simulink model "Quad_UAV_Dynamics"  (R2024b)
settings: Solver=ode4  StartTime=0.0  StopTime=inf  FixedStep=SampleTime  RelTol=1e-3
PreLoadFcn:
  | InitVars;
undefined symbols (not defined in the file): contact, control, Controller, Defectiveness, Environment, Estimator, fractalcoef, m_to_mm, ms2_to_mg, ms_to_cms, Payload, ref_height, ref_lat, ref_lon, rotorDir, rotorPositions, rotorThrustMax, rotorTimeConst, rotorTorqueMax, SampleTime, SampleTimePlant, SamplingTime, Vehicle
libraries: slpidlib x9, uavmavlinklib x9, simulink_extras x3, simulink x2, sharedtransform x2, aerolibatmos2 x1, sensorgpslib x1, robotcorelib x1, mspsensorlib x1, shared6dof x1, aerolibasang x1, sldrtlib x1
(part 2 of 2)

== system Quad_UAV_Dynamics/Send Plant Feedback/HIL_QUATERNION ==
  Acc : Inport
  States : Inport  Port=2
  GPS Subsystem : Subsystem
      settings: PortSchema="{\"entries\":[{\"content\":{\"sides\":[{\"content\":{\"connectorIds\":[\"In1\"]},\"type\":\"ConnectorPlacement.EquallySpacedRectSide\",\"uuid\":\"bd7d303d-974a-4dd9-8d27-04cf87176bd7\"},{\"content\":{\"connectorIds\":[\"Out1\"],\"side\":\"RIGHT\"},\"type\":\"ConnectorPlacement.EquallySpacedRectSide\",\"uuid\":\"9b60b4cf-af27-4ca7-86b7-e75d27668f15\"},{\"content\":{\"connectorIds\":[\"In2\"],\"side\":\"TOP\"},\"type\":\"ConnectorPlacement.EquallySpacedRectSide\",\"uuid\":\"cd4d20a6-3033-4c65-942d-f02a7fa933e8\"},{\"content\":{\"side\":\"BOTTOM\"},\"type\":\"ConnectorPlacement.EquallySpacedRectSide\",\"uuid\":\"d837ff15-3ee7-4ba9-aab0-0378a7633b3a\"},{\"content\":{\"side\":\"HIDDEN\"},\"type\":\"ConnectorPlacement.EquallySpacedRectSide\",\"uuid\":\"eefe2c49-f98f-4c11-8e75-b071b558b610\"}]},\"type\":\"ConnectorPlacement.EquallySpacedConnector\",\"uuid\":\"bd9fca06-cb18-49af-bec9-4d4823ab7b04\"}],\"packageUris\":[\"http://schema.mathworks.com/mf0/Connector/R2020b\"],\"version\":\"1.0\"}"
  MAVLink Serializer2 : uavmavlinklib/MAVLink Serializer  dialectSource=Select from standard MAVLink dialects  dialect=common.xml  dialectCustom=common.xml  version=2  messageType=HIL_STATE_QUATERNION
  Terminator2 : Terminator
  HIL_QUATERNION_bytes : Outport
  wires:
  States/1 -> GPS Subsystem/1(States)
  MAVLink Serializer2/2 -> Terminator2/1
  GPS Subsystem/1(HIL Quaternion) -> MAVLink Serializer2/1
  MAVLink Serializer2/1 -> HIL_QUATERNION_bytes/1
  Acc/1 -> GPS Subsystem/2(Acc)

== system Quad_UAV_Dynamics/Send Plant Feedback/HIL_SENSOR ==
  Acc : Inport
  Gyro : Inport  Port=2
  Mag : Inport  Port=3
  Pressure : Inport  Port=4
  Hil Sensor Creation subsystem : Subsystem
  MAVLink Serializer1 : uavmavlinklib/MAVLink Serializer  dialectSource=Select from standard MAVLink dialects  dialect=common.xml  dialectCustom=common.xml  version=2  messageType=HIL_SENSOR
  Terminator1 : Terminator
  HIL_SENSOR_bytes : Outport
  wires:
  MAVLink Serializer1/2 -> Terminator1/1
  Hil Sensor Creation subsystem/1(HIL Sensor) -> MAVLink Serializer1/1
  Acc/1 -> Hil Sensor Creation subsystem/1(Acc)
  MAVLink Serializer1/1 -> HIL_SENSOR_bytes/1
  Gyro/1 -> Hil Sensor Creation subsystem/2(Gyro)
  Mag/1 -> Hil Sensor Creation subsystem/3(Mag)
  Pressure/1 -> Hil Sensor Creation subsystem/4(Pressure)

== system Quad_UAV_Dynamics/Send Plant Feedback/Send Heartbeat ==
  Bus Assignment : BusAssignment  AssignedSignals=Payload.autopilot,Payload.type
  Constant : Constant  SampleTime=-1
  Constant1 : Constant  Value=12  SampleTime=-1
  Data Type Conversion : DataTypeConversion  OutDataTypeStr=uint8  SaturateOnIntegerOverflow=off  RndMeth=Floor
  Data Type Conversion1 : DataTypeConversion  OutDataTypeStr=uint8  SaturateOnIntegerOverflow=off  RndMeth=Floor
  MAVLink Blank Message : uavmavlinklib/MAVLink Blank Message  dialectSource=Select from standard MAVLink dialects  dialect=common.xml  dialectCustom=common.xml  version=2  messageType=HEARTBEAT  SystemID=2  ComponentID=51  SampleTime=SampleTime
  MAVLink Serializer : uavmavlinklib/MAVLink Serializer  dialectSource=Select from standard MAVLink dialects  dialect=common.xml  dialectCustom=common.xml  version=2  messageType=HEARTBEAT
  Terminator4 : Terminator
  HEARTBEAT_bytes : Outport
  wires:
  Bus Assignment/1 -> MAVLink Serializer/1
  Constant/1 -> Data Type Conversion/1
  MAVLink Serializer/1 -> HEARTBEAT_bytes/1
  Data Type Conversion1/1 -> Bus Assignment/3
  Data Type Conversion/1 -> Bus Assignment/2
  MAVLink Serializer/2 -> Terminator4/1
  Constant1/1 -> Data Type Conversion1/1
  MAVLink Blank Message/1 -> Bus Assignment/1

== system Quad_UAV_Dynamics/Plant/IMU Simulation/IMU Subsystem ==
  States : Inport
  Bus Selector1 : BusSelector  OutputSignals=p,q,r  OutputAsBus=on
  Bus Selector2 : BusSelector  OutputSignals=yaw,pitch,roll  OutputAsBus=on
  Bus Selector3 : BusSelector  OutputSignals=ddx,ddy,ddz  OutputAsBus=on
  Coordinate Transformation Conversion1 : robotcorelib/Coordinate Transformation Conversion  InputRepresentation=Euler Angles  InputEulerSequence=ZYX  ShowTrVecInputPort=on  OutputRepresentation=Quaternion  OutputEulerSequence=ZYX  ShowTrVecOutputPort=on  SimulateUsing=Interpreted execution
  Gain : Gain  Gain=-1
  IMU : mspsensorlib/IMU  DispRefFrame=NED  TemperaturePort=off  Temperature=25  MagneticFieldPort=off  MagneticFieldNED=[ 27.5550, -2.4169, -16.0849 ]  MagneticFieldENU=[ -2.4169, 27.5550, 16.0849 ]  SeedDouble=67  SimulateUsing=Interpreted execution  AccelParamsMeasurementRange=Inf  AccelParamsResolution=0  AccelParamsConstantBias=[ 0, 0, 0 ]  AccelParamsAxesMisalignment=[ 0, 0, 0 ]  AccelParamsNoiseDensity=[ 0, 0, 0 ]  AccelParamsBiasInstability=[ 0, 0, 0 ]  AccelParamsBiasInstabilityNumerator=fractalcoef().Numerator  AccelParamsBiasInstabilityDenominator=fractalcoef().Denominator  AccelParamsRandomWalk=[ 0, 0, 0 ]  AccelParamsNoiseType=double-sided  AccelParamsTemperatureBias=[ 0, 0, 0 ]  AccelParamsTemperatureScaleFactor=[ 0, 0, 0 ]  GyroParamsMeasurementRange=Inf  GyroParamsResolution=0  GyroParamsConstantBias=[ 0, 0, 0 ]  GyroParamsAxesMisalignment=[ 0, 0, 0 ]  GyroParamsAccelerationBias=[ 0, 0, 0 ]  GyroParamsNoiseDensity=[ 0, 0, 0 ]  GyroParamsBiasInstability=[ 0, 0, 0 ]  GyroParamsBiasInstabilityNumerator=fractalcoef().Numerator  GyroParamsBiasInstabilityDenominator=fractalcoef().Denominator  GyroParamsRandomWalk=[ 0, 0, 0 ]  GyroParamsNoiseType=double-sided  GyroParamsTemperatureBias=[ 0, 0, 0 ]  GyroParamsTemperatureScaleFactor=[ 0, 0, 0 ]  MagParamsMeasurementRange=Inf  MagParamsResolution=0  MagParamsConstantBias=[ 0, 0, 0 ]  MagParamsAxesMisalignment=[ 0, 0, 0 ]  MagParamsNoiseDensity=[ 0, 0, 0 ]  MagParamsBiasInstability=[ 0, 0, 0 ]  MagParamsBiasInstabilityNumerator=fractalcoef().Numerator  MagParamsBiasInstabilityDenominator=fractalcoef().Denominator  MagParamsRandomWalk=[ 0, 0, 0 ]  MagParamsNoiseType=double-sided  MagParamsTemperatureBias=[ 0, 0, 0 ]  MagParamsTemperatureScaleFactor=[ 0, 0, 0 ]
  Reshape : Reshape  OutputDimensionality=Row vector (2-D)
  Reshape2 : Reshape  OutputDimensionality=Row vector (2-D)
  Reshape3 : Reshape  OutputDimensionality=Row vector (2-D)
  Acc : Outport
  Gyro : Outport  Port=2
  Mag : Outport  Port=3
  wires:
  Bus Selector1/1 -> Reshape2/1
  IMU/1 -> Gain/1
  Bus Selector2/1 -> Coordinate Transformation Conversion1/1
  IMU/3 -> Mag/1
  Reshape2/1 -> IMU/2
  Bus Selector3/1 -> Reshape/1
  Coordinate Transformation Conversion1/1 -> Reshape3/1
  Reshape/1 -> IMU/1
  IMU/2 -> Gyro/1
  Reshape3/1 -> IMU/3
  States/1 -> Bus Selector3/1, Bus Selector2/1, Bus Selector1/1
  Gain/1 -> Acc/1

== system Quad_UAV_Dynamics/Plant/Non-Linear Airframe/AC model ==
  Actuators : Inport
  States : Inport  Port=2
  Add1 : Sum  Inputs=++++
  Add2 : Sum  Inputs=+++
  Aerodynamic : Subsystem
  Bus Selector3 : BusSelector  OutputSignals=DCM
  Constant : Constant  Value=Environment.g
  Constant1 : Constant  Value=Environment.rho
  Gravity Force Calculation : Subsystem
  Ground Model : Subsystem
  Motor Forces and Torques : Subsystem
  Rotor Model : Subsystem  Commented=on
  F_cg : Outport  Unit=N  VectorParamsAs1DForOutWhenUnconnected=off
  M_cg : Outport  Port=2  Unit=N*m  VectorParamsAs1DForOutWhenUnconnected=off
  wires:
  Add1/1 -> F_cg/1
  Constant/1 -> Gravity Force Calculation/2(gravity)
  Constant1/1 -> Aerodynamic/1(Density)
  States/1 -> Bus Selector3/1, Ground Model/1(States), Aerodynamic/2(States)
  Actuators/1 -> Motor Forces and Torques/1(Input [0-1])
  Bus Selector3/1 -> Gravity Force Calculation/1(DCMbe)  "<DCM>"
  Add2/1 -> M_cg/1
  Motor Forces and Torques/2(Motor Torques) -> Add2/2
  Motor Forces and Torques/1(Motor Forces) -> Add1/3
  Gravity Force Calculation/1(gravity force) -> Add1/1
  Aerodynamic/2(Moment) -> Add2/1
  Aerodynamic/1(Force) -> Add1/2
  Ground Model/1(Fb_contact) -> Add1/4
  Ground Model/2(Mb_contact) -> Add2/3

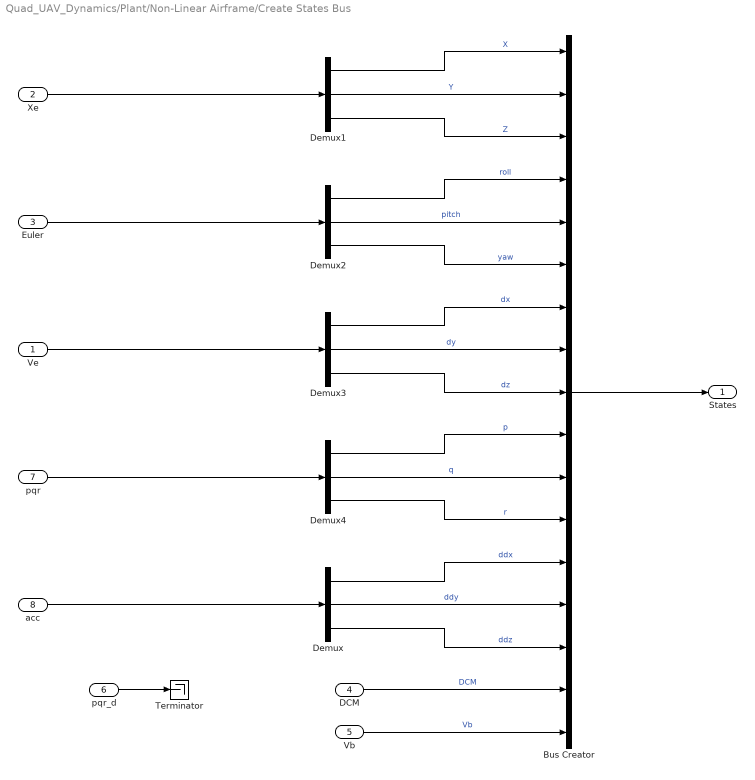
== system Quad_UAV_Dynamics/Plant/Non-Linear Airframe/Create States Bus ==
  Ve : Inport
  Xe : Inport  Port=2
  Euler : Inport  Port=3
  DCM : Inport  Port=4
  Vb : Inport  Port=5
  pqr_d : Inport  Port=6
  pqr : Inport  Port=7
  acc : Inport  Port=8
  Bus Creator : BusCreator  Inputs=17
  Demux{,1..4} (5 alike) : Demux  Outputs=3
  Terminator : Terminator
  States : Outport
  wires:
  Demux1/1 -> Bus Creator/1  "X"
  Demux1/2 -> Bus Creator/2  "Y"
  Euler/1 -> Demux2/1
  Demux2/2 -> Bus Creator/5  "pitch"
  Demux3/2 -> Bus Creator/8  "dy"
  Demux2/3 -> Bus Creator/6  "yaw"
  pqr/1 -> Demux4/1
  Ve/1 -> Demux3/1
  Demux2/1 -> Bus Creator/4  "roll"
  Demux1/3 -> Bus Creator/3  "Z"
  Demux3/1 -> Bus Creator/7  "dx"
  Demux4/2 -> Bus Creator/11  "q"
  Demux3/3 -> Bus Creator/9  "dz"
  Demux4/3 -> Bus Creator/12  "r"
  Demux4/1 -> Bus Creator/10  "p"
  Bus Creator/1 -> States/1
  Xe/1 -> Demux1/1
  acc/1 -> Demux/1
  Demux/3 -> Bus Creator/15  "ddz"
  Demux/2 -> Bus Creator/14  "ddy"
  Demux/1 -> Bus Creator/13  "ddx"
  DCM/1 -> Bus Creator/16  "DCM"
  Vb/1 -> Bus Creator/17  "Vb"
  pqr_d/1 -> Terminator/1

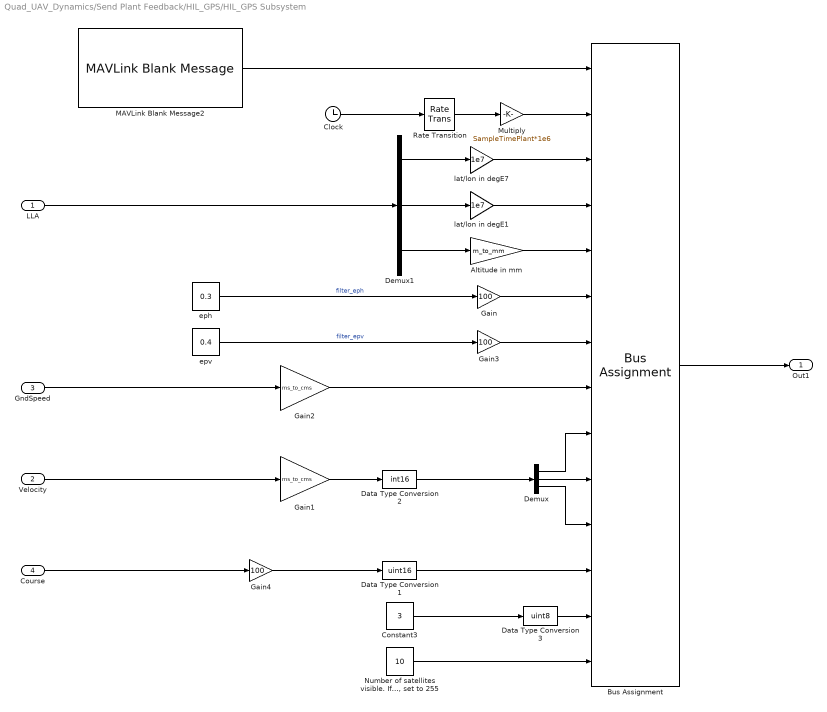
== system Quad_UAV_Dynamics/Send Plant Feedback/HIL_GPS/HIL_GPS Subsystem ==
  LLA : Inport
  Velocity : Inport  Port=2
  GndSpeed : Inport  Port=3
  Course : Inport  Port=4
  Altitude in mm : Gain  Gain=m_to_mm  OutDataTypeStr=Inherit: Inherit via back propagation
  Bus Assignment : BusAssignment  AssignedSignals=Payload.time_usec,Payload.lat,Payload.lon,Payload.alt,Payload.eph,Payload.epv,Payload.vel,Payload.vn,Payload.ve,Payload.vd,Payload.cog,Payload.fix_type,Payload.satellites_visible
  Clock : Clock
  Constant3 : Constant  Value=3  OutDataTypeStr=Inherit: Inherit via back propagation  SampleTime=-1
  Data Type Conversion1 : DataTypeConversion  OutDataTypeStr=uint16  SaturateOnIntegerOverflow=off  RndMeth=Floor
  Data Type Conversion2 : DataTypeConversion  OutDataTypeStr=int16  SaturateOnIntegerOverflow=off  RndMeth=Floor
  Data Type Conversion3 : DataTypeConversion  OutDataTypeStr=uint8  SaturateOnIntegerOverflow=off  RndMeth=Floor
  Demux : Demux  Outputs=3
  Demux1 : Demux  Outputs=3
  Gain : Gain  Gain=100  OutDataTypeStr=Inherit: Inherit via back propagation
  Gain1 : Gain  Gain=ms_to_cms
  Gain2 : Gain  Gain=ms_to_cms  OutDataTypeStr=uint16
  Gain3 : Gain  Gain=100  OutDataTypeStr=Inherit: Inherit via back propagation
  Gain4 : Gain  Gain=100
  MAVLink Blank Message2 : uavmavlinklib/MAVLink Blank Message  dialectSource=Select from standard MAVLink dialects  dialect=common.xml  dialectCustom=common.xml  version=2  messageType=HIL_GPS  SystemID=2  ComponentID=51  SampleTime=SampleTime
  Multiply : Gain  Gain=SampleTimePlant*1e6  OutDataTypeStr=Inherit: Inherit via back propagation
  "Number of satellites visible. If unknown, set to 255" : Constant  Value=10  OutDataTypeStr=Inherit: Inherit via back propagation  SampleTime=-1
  Rate Transition : RateTransition
  eph : Constant  Value=0.3  SampleTime=-1
  epv : Constant  Value=0.4  SampleTime=-1
  lat/lon in degE1 : Gain  Gain=1e7  OutDataTypeStr=Inherit: Inherit via back propagation
  lat/lon in degE7 : Gain  Gain=1e7  OutDataTypeStr=Inherit: Inherit via back propagation
  Out1 : Outport
  wires:
  Gain2/1 -> Bus Assignment/8
  lat/lon in degE7/1 -> Bus Assignment/3
  Demux1/1 -> lat/lon in degE7/1
  Demux/3 -> Bus Assignment/11
  MAVLink Blank Message2/1 -> Bus Assignment/1
  Gain1/1 -> Data Type Conversion2/1
  Demux1/3 -> Altitude in mm/1
  Demux1/2 -> lat/lon in degE1/1
  Demux/1 -> Bus Assignment/9
  lat/lon in degE1/1 -> Bus Assignment/4
  Altitude in mm/1 -> Bus Assignment/5
  Data Type Conversion2/1 -> Demux/1
  Demux/2 -> Bus Assignment/10
  Bus Assignment/1 -> Out1/1
  "Number of satellites visible. If unknown, set to 255"/1 -> Bus Assignment/14
  Gain/1 -> Bus Assignment/6
  Gain3/1 -> Bus Assignment/7
  LLA/1 -> Demux1/1
  GndSpeed/1 -> Gain2/1
  Velocity/1 -> Gain1/1
  Course/1 -> Gain4/1
  Data Type Conversion1/1 -> Bus Assignment/12
  eph/1 -> Gain/1  "filter_eph"
  epv/1 -> Gain3/1  "filter_epv"
  Data Type Conversion3/1 -> Bus Assignment/13
  Gain4/1 -> Data Type Conversion1/1
  Constant3/1 -> Data Type Conversion3/1
  Clock/1 -> Rate Transition/1
  Rate Transition/1 -> Multiply/1
  Multiply/1 -> Bus Assignment/2

== system Quad_UAV_Dynamics/Send Plant Feedback/HIL_QUATERNION/GPS Subsystem ==
  States : Inport
  Acc : Inport  Port=2
  HIL Quaternion Creation Subsystem : Subsystem
  HIL Quaternion : Outport
  wires:
  HIL Quaternion Creation Subsystem/1(HIL Quaternion) -> HIL Quaternion/1
  States/1 -> HIL Quaternion Creation Subsystem/2(States)
  Acc/1 -> HIL Quaternion Creation Subsystem/1(Acc)

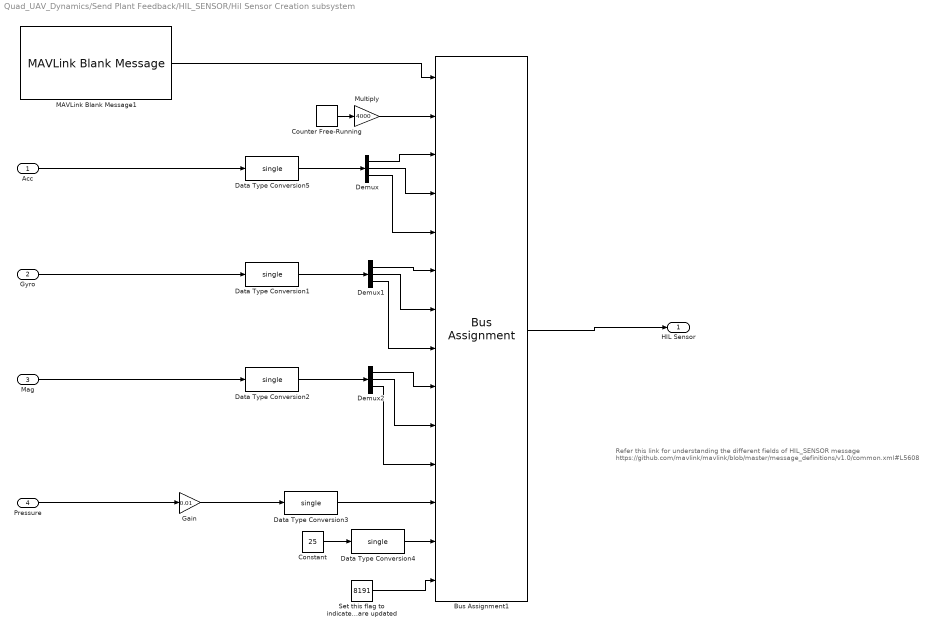
== system Quad_UAV_Dynamics/Send Plant Feedback/HIL_SENSOR/Hil Sensor Creation subsystem ==
  note: Refer this link for understanding the different fields of HIL_SENSOR message https://github.com/mavlink/mavlink/blob/master/message_definitions/v1.0/common.xml#L5608
  Acc : Inport
  Gyro : Inport  Port=2
  Mag : Inport  Port=3
  Pressure : Inport  Port=4
  Bus Assignment1 : BusAssignment  AssignedSignals=Payload.time_usec,Payload.xacc,Payload.yacc,Payload.zacc,Payload.xgyro,Payload.ygyro,Payload.zgyro,Payload.xmag,Payload.ymag,Payload.zmag,Payload.abs_pressure,Payload.temperature,Payload.fields_updated
  Constant : Constant  Value=25
  Counter Free-Running : simulink/Sources/Counter Free-Running  NumBits=64  tsamp=SampleTime
  Data Type Conversion{1..5} (5 alike) : DataTypeConversion  OutDataTypeStr=single  SaturateOnIntegerOverflow=off  RndMeth=Floor
  Demux : Demux  Outputs=3
  Demux1 : Demux  Outputs=3
  Demux2 : Demux  Outputs=3
  Gain : Gain  Gain=0.01
  MAVLink Blank Message1 : uavmavlinklib/MAVLink Blank Message  dialectSource=Select from standard MAVLink dialects  dialect=common.xml  dialectCustom=common.xml  version=2  messageType=HIL_SENSOR  SystemID=2  ComponentID=51  SampleTime=SampleTime
  Multiply : Gain  Gain=4000  OutDataTypeStr=Inherit: Inherit via back propagation
  Set this flag to indicate all flags are updated : Constant  Value=8191  OutDataTypeStr=Inherit: Inherit via back propagation  SampleTime=-1
  HIL Sensor : Outport
  wires:
  Data Type Conversion2/1 -> Demux2/1
  Demux1/1 -> Bus Assignment1/6
  Counter Free-Running/1 -> Multiply/1
  Demux1/3 -> Bus Assignment1/8
  Data Type Conversion1/1 -> Demux1/1
  Gyro/1 -> Data Type Conversion1/1
  Bus Assignment1/1 -> HIL Sensor/1
  Set this flag to indicate all flags are updated/1 -> Bus Assignment1/14
  Demux/3 -> Bus Assignment1/5
  Demux2/2 -> Bus Assignment1/10
  Demux2/3 -> Bus Assignment1/11
  Data Type Conversion5/1 -> Demux/1
  Demux/1 -> Bus Assignment1/3
  MAVLink Blank Message1/1 -> Bus Assignment1/1
  Demux2/1 -> Bus Assignment1/9
  Demux/2 -> Bus Assignment1/4
  Demux1/2 -> Bus Assignment1/7
  Acc/1 -> Data Type Conversion5/1
  Mag/1 -> Data Type Conversion2/1
  Data Type Conversion3/1 -> Bus Assignment1/12
  Gain/1 -> Data Type Conversion3/1
  Pressure/1 -> Gain/1
  Constant/1 -> Data Type Conversion4/1
  Data Type Conversion4/1 -> Bus Assignment1/13
  Multiply/1 -> Bus Assignment1/2

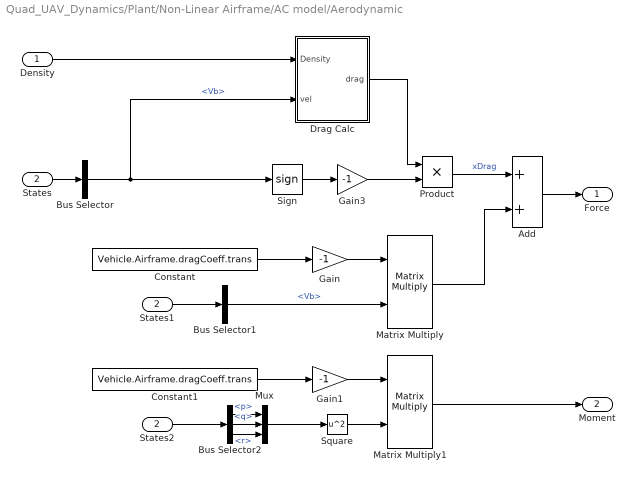
== system Quad_UAV_Dynamics/Plant/Non-Linear Airframe/AC model/Aerodynamic ==
  Density : Inport  Unit=kg/m^3
  States : Inport  Port=2
  Add : Sum
  Bus Selector : BusSelector  OutputSignals=Vb
  Bus Selector1 : BusSelector  OutputSignals=Vb
  Bus Selector2 : BusSelector  OutputSignals=p,q,r
  Constant : Constant  Value=Vehicle.Airframe.dragCoeff.trans
  Constant1 : Constant  Value=Vehicle.Airframe.dragCoeff.trans
  Drag Calc : Subsystem
  Gain : Gain  Gain=-1
  Gain1 : Gain  Gain=-1
  Gain3 : Gain  Gain=-1
  Matrix Multiply : Product  Multiplication=Matrix(*)
  Matrix Multiply1 : Product  Multiplication=Matrix(*)
  Mux : Mux  Inputs=3
  Product : Product  RndMeth=Zero
  Sign : Signum  ZeroCross=off
  Square : Math  Operator=square
  States1 : InportShadow  Port=2
  States2 : InportShadow  Port=2
  Force : Outport  Unit=N  VectorParamsAs1DForOutWhenUnconnected=off
  Moment : Outport  Port=2  Unit=N  VectorParamsAs1DForOutWhenUnconnected=off
  wires:
  Density/1 -> Drag Calc/1(Density)
  Sign/1 -> Gain3/1
  Drag Calc/1(drag) -> Product/1
  Product/1 -> Add/1  "xDrag"
  Bus Selector/1 -> Drag Calc/2(vel), Sign/1  "<Vb>"
  Gain3/1 -> Product/2
  States/1 -> Bus Selector/1
  Constant/1 -> Gain/1
  States1/1 -> Bus Selector1/1
  Bus Selector1/1 -> Matrix Multiply/2  "<Vb>"
  Matrix Multiply/1 -> Add/2
  Add/1 -> Force/1
  Constant1/1 -> Gain1/1
  States2/1 -> Bus Selector2/1
  Gain/1 -> Matrix Multiply/1
  Gain1/1 -> Matrix Multiply1/1
  Square/1 -> Matrix Multiply1/2
  Matrix Multiply1/1 -> Moment/1
  Bus Selector2/1 -> Mux/1  "<p>"
  Bus Selector2/2 -> Mux/2  "<q>"
  Bus Selector2/3 -> Mux/3  "<r>"
  Mux/1 -> Square/1

== system Quad_UAV_Dynamics/Plant/Non-Linear Airframe/AC model/Gravity Force Calculation ==
  DCMbe : Inport
  gravity : Inport  Port=2  Unit=m/s^2
  Gain1 : Gain  Gain=Vehicle.Airframe.mass
  Product : Product  Multiplication=Matrix(*)
  gravity force : Outport  Unit=N  VectorParamsAs1DForOutWhenUnconnected=off
  wires:
  gravity/1 -> Gain1/1
  Gain1/1 -> Product/2  "gravity force NED"
  Product/1 -> gravity force/1
  DCMbe/1 -> Product/1

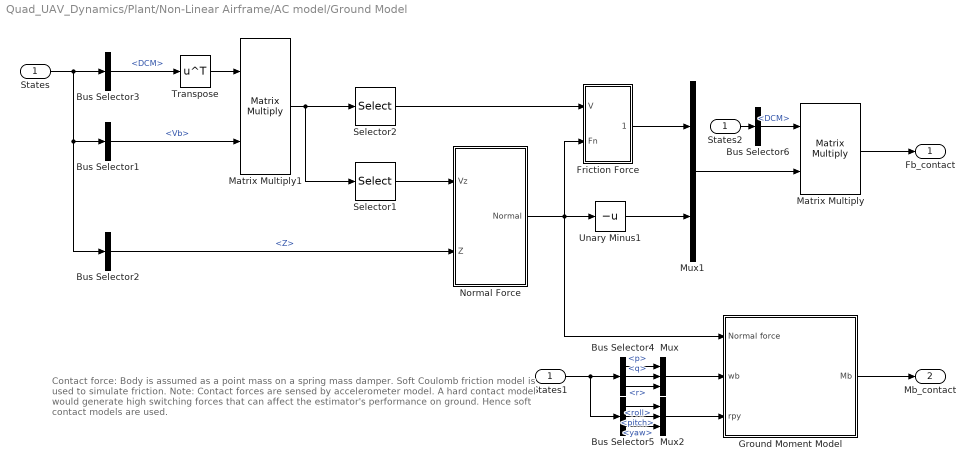
== system Quad_UAV_Dynamics/Plant/Non-Linear Airframe/AC model/Ground Model ==
  note: Contact force:
      | Body is assumed as a point mass on a spring mass damper. Soft Coulomb friction model is used to simulate friction.
      |
      | Note:
      | Contact forces are sensed by accelerometer model. A hard contact model would generate high switching forces that can affect the estimator's performance on ground. Hence soft contact models are used.
  States : Inport
  Bus Selector1 : BusSelector  OutputSignals=Vb
  Bus Selector2 : BusSelector  OutputSignals=Z
  Bus Selector3 : BusSelector  OutputSignals=DCM
  Bus Selector4 : BusSelector  OutputSignals=p,q,r
  Bus Selector5 : BusSelector  OutputSignals=roll,pitch,yaw
  Bus Selector6 : BusSelector  OutputSignals=DCM
  Friction Force : Subsystem
  Ground Moment Model : Subsystem
  Matrix Multiply : Product  Multiplication=Matrix(*)
  Matrix Multiply1 : Product  Multiplication=Matrix(*)
  Mux : Mux  Inputs=3
  Mux1 : Mux  Inputs=2
  Mux2 : Mux  Inputs=3
  Normal Force : Subsystem
  Selector1 : Selector  InputPortWidth=3  IndexOptions=Index vector (dialog)  Indices=[3]  OutputSizes=1
  Selector2 : Selector  InputPortWidth=3  IndexOptions=Index vector (dialog)  Indices=[1,2]  OutputSizes=1
  States1 : InportShadow
  States2 : InportShadow
  Transpose : Math  Operator=transpose
  Unary Minus1 : UnaryMinus
  Fb_contact : Outport
  Mb_contact : Outport  Port=2
  wires:
  Selector1/1 -> Normal Force/1(Vz)
  Bus Selector2/1 -> Normal Force/2(Z)  "<Z>"
  Matrix Multiply/1 -> Fb_contact/1
  Normal Force/1(Normal) -> Unary Minus1/1, Ground Moment Model/1(Normal force), Friction Force/2(Fn)
  Mux1/1 -> Matrix Multiply/2
  Unary Minus1/1 -> Mux1/2
  Selector2/1 -> Friction Force/1(V)
  Friction Force/1(Friction) -> Mux1/1
  Bus Selector3/1 -> Transpose/1  "<DCM>"
  Transpose/1 -> Matrix Multiply1/1
  Bus Selector1/1 -> Matrix Multiply1/2  "<Vb>"
  Matrix Multiply1/1 -> Selector1/1, Selector2/1
  Ground Moment Model/1(Mb) -> Mb_contact/1
  States/1 -> Bus Selector3/1, Bus Selector1/1, Bus Selector2/1
  States1/1 -> Bus Selector4/1, Bus Selector5/1
  Bus Selector4/1 -> Mux/1  "<p>"
  Bus Selector4/2 -> Mux/2  "<q>"
  Bus Selector4/3 -> Mux/3  "<r>"
  Mux/1 -> Ground Moment Model/2(wb)
  Bus Selector5/1 -> Mux2/1  "<roll>"
  Bus Selector5/2 -> Mux2/2  "<pitch>"
  Bus Selector5/3 -> Mux2/3  "<yaw>"
  Mux2/1 -> Ground Moment Model/3(rpy)
  States2/1 -> Bus Selector6/1
  Bus Selector6/1 -> Matrix Multiply/1  "<DCM>"

== system Quad_UAV_Dynamics/Plant/Non-Linear Airframe/AC model/Motor Forces and Torques ==
  Input [0-1] : Inport
  Add : Sum
  Deffectiveness : Subsystem  Commented=on  mask(Control Signal Mapper){d1=Defectiveness.Actuator_1.value, d2=Defectiveness.Actuator_2.value, d3=Defectiveness.Actuator_3.value, d4=Defectiveness.Actuator_4.value, d1_start=Defectiveness.Actuator_1.StartTime, d1_stop=Defectiveness.Actuator_1.endTime, d2_start=Defectiveness.Actuator_2.StartTime, d2_stop=Defectiveness.Actuator_2.endTime, d3_start=Defectiveness.Actuator_3.StartTime, d3_stop=Defectiveness.Actuator_3.endTime, d4_start=Defectiveness.Actuator_4.StartTime, d4_stop=Defectiveness.Actuator_4.endTime}
      mask prompts: d1 "Actuator-1"; d2 "Actuator-2"; d3 "Actuator-3"; d4 "Actuator-4"; d1_start "Start"; d1_stop "Stop"; d2_start "Start"; d2_stop "Stop"; d3_start "Start"; d3_stop "Stop"; d4_start "Start"; d4_stop "Stop"
      mask help:
      | This block maps control signals to each actuator. This block also generates a desired defectiveness value at specified start and stop time.
      |
      | Minimum and maximum defectiveness values are 0 and 1 respectively.
      settings: MinAlgLoopOccurrences=on
      mask Help: Should user exceeds the max or min value the limitation will correct it.
      mask DialogControl ParameterGroupVar Prompt: Defectiveness Values
      mask DialogControl Container4 Prompt: Defectiveness Time
      mask DialogControl Container5 Prompt: Actuator - 1
      mask DialogControl Container6 Prompt: Actuator - 2
      mask DialogControl Container8 Prompt: Actuator - 3
      mask DialogControl Container9 Prompt: Actuator - 4
  Gain2 : Gain  Gain=-1
  Gyroscopic Moments : Subsystem
  Mapper : Constant  Value=Controller.motorMapper  OutDataTypeStr=double
  Motor : Subsystem
  Mux : Mux  Inputs=3
  Product : Product  Multiplication=Matrix(*)  RndMeth=Zero
  Selector : Selector  InputPortWidth=4  IndexOptions=Index vector (dialog)  Indices=1  OutputSizes=1
  Selector1 : Selector  InputPortWidth=4  IndexOptions=Index vector (dialog)  Indices=2:4  OutputSizes=1
  Square : Math  Operator=square
  Zero : Constant  Value=0  OutDataTypeStr=Inherit: Inherit via back propagation
  Motor Forces : Outport  OutDataTypeStr=double  Unit=N  PortDimensions=3  SampleTime=0  VectorParamsAs1DForOutWhenUnconnected=off
  Motor Torques : Outport  Port=2  OutDataTypeStr=double  Unit=N*m  PortDimensions=3  SampleTime=0  VectorParamsAs1DForOutWhenUnconnected=off
  wires:
  Square/1 -> Product/2
  Gyroscopic Moments/1(M) -> Add/2
  Add/1 -> Motor Torques/1
  Motor/1(rpm) -> Square/1, Gyroscopic Moments/1(Omega)
  Input [0-1]/1 -> Motor/1(PWM)
  Product/1 -> Selector1/1, Selector/1
  Gain2/1 -> Motor Forces/1
  Selector/1 -> Mux/3
  Mapper/1 -> Product/1
  Selector1/1 -> Add/1
  Mux/1 -> Gain2/1
  Zero/1 -> Mux/2, Mux/1

== system Quad_UAV_Dynamics/Plant/Non-Linear Airframe/AC model/Rotor Model ==
  Input [0-1] : Inport
  Constant : Constant  Value=rotorPositions
  Constant1 : Constant  Value=rotorDir
  MATLAB Function : MATLAB Function  TreatAsAtomicUnit=on
  Thrust model : Subsystem
  Torque model : Subsystem
  F_rotors : Outport
  M_rotors : Outport  Port=2
  wires:
  Input [0-1]/1 -> Torque model/1(In1), Thrust model/1(In1)
  MATLAB Function/1(netF) -> F_rotors/1
  MATLAB Function/2(netM) -> M_rotors/1
  Constant/1 -> MATLAB Function/3(rotorPositions)
  Constant1/1 -> MATLAB Function/4(rotorDir)
  Torque model/1(Out1) -> MATLAB Function/2(tauEachRotor)
  Thrust model/1(Out1) -> MATLAB Function/1(thrustEachRotor)

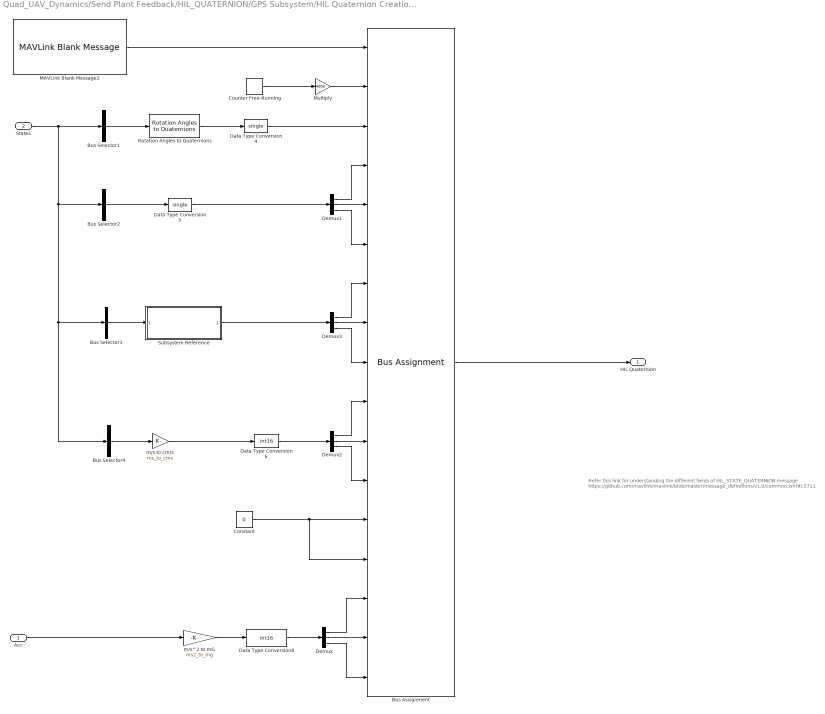
== system Quad_UAV_Dynamics/Send Plant Feedback/HIL_QUATERNION/GPS Subsystem/HIL Quaternion Creation Subsystem ==
  note: Refer this link for understanding the different fields of HIL_STATE_QUATERNION message https://github.com/mavlink/mavlink/blob/master/message_definitions/v1.0/common.xml#L5711
  Acc : Inport
  States : Inport  Port=2
  Bus Assignment : BusAssignment  AssignedSignals=Payload.time_usec,Payload.attitude_quaternion,Payload.rollspeed,Payload.pitchspeed,Payload.yawspeed,Payload.lat,Payload.lon,Payload.alt,Payload.vx,Payload.vy,Payload.vz,Payload.ind_airspeed,Payload.true_airspeed,Payload.xacc,Payload.yacc,Payload.zacc
  Bus Selector1 : BusSelector  OutputSignals=yaw,pitch,roll  OutputAsBus=on
  Bus Selector2 : BusSelector  OutputSignals=r,q,p  OutputAsBus=on
  Bus Selector3 : BusSelector  OutputSignals=X,Y,Z  OutputAsBus=on
  Bus Selector4 : BusSelector  OutputSignals=dx,dy,dz  OutputAsBus=on
  Constant : Constant  Value=0  OutDataTypeStr=Inherit: Inherit via back propagation
  Counter Free-Running : simulink/Sources/Counter Free-Running  NumBits=64  tsamp=-1
  Data Type Conversion4 : DataTypeConversion  OutDataTypeStr=single  SaturateOnIntegerOverflow=off  RndMeth=Floor
  Data Type Conversion5 : DataTypeConversion  OutDataTypeStr=single  SaturateOnIntegerOverflow=off  RndMeth=Floor
  Data Type Conversion6 : DataTypeConversion  OutDataTypeStr=int16  SaturateOnIntegerOverflow=off  RndMeth=Floor
  Data Type Conversion8 : DataTypeConversion  OutDataTypeStr=int16  SaturateOnIntegerOverflow=off  RndMeth=Floor
  Demux{,1..3} (4 alike) : Demux  Outputs=3
  MAVLink Blank Message2 : uavmavlinklib/MAVLink Blank Message  dialectSource=Select from standard MAVLink dialects  dialect=common.xml  dialectCustom=common.xml  version=2  messageType=HIL_STATE_QUATERNION  SystemID=2  ComponentID=51  SampleTime=SampleTime
  Multiply : Gain  Gain=4000  OutDataTypeStr=Inherit: Inherit via back propagation
  Rotation Angles to Quaternions : sharedtransform/Rotation Angles to Quaternions  rotationOrder=ZYX  aMode=aMode
  Subsystem Reference : Subsystem  ReferencedSubsystem=Create_LLA_from_States
  m/s to cm/s : Gain  Gain=ms_to_cms
  m/s^2 to mG : Gain  Gain=ms2_to_mg
  HIL Quaternion : Outport
  wires:
  Counter Free-Running/1 -> Multiply/1
  MAVLink Blank Message2/1 -> Bus Assignment/1
  Multiply/1 -> Bus Assignment/2
  Bus Assignment/1 -> HIL Quaternion/1
  States/1 -> Bus Selector1/1, Bus Selector2/1, Bus Selector4/1, Bus Selector3/1
  Rotation Angles to Quaternions/1 -> Data Type Conversion4/1
  Data Type Conversion4/1 -> Bus Assignment/3
  Demux/3 -> Bus Assignment/17
  Demux/1 -> Bus Assignment/15
  Demux/2 -> Bus Assignment/16
  Constant/1 -> Bus Assignment/14, Bus Assignment/13
  m/s to cm/s/1 -> Data Type Conversion6/1
  Data Type Conversion6/1 -> Demux2/1
  Demux2/3 -> Bus Assignment/12
  Demux2/2 -> Bus Assignment/11
  Demux2/1 -> Bus Assignment/10
  Subsystem Reference/1 -> Demux3/1
  Demux3/1 -> Bus Assignment/7
  Demux3/2 -> Bus Assignment/8
  Demux3/3 -> Bus Assignment/9
  Data Type Conversion8/1 -> Demux/1
  Acc/1 -> m/s^2 to mG/1
  m/s^2 to mG/1 -> Data Type Conversion8/1
  Bus Selector1/1 -> Rotation Angles to Quaternions/1
  Data Type Conversion5/1 -> Demux1/1
  Demux1/3 -> Bus Assignment/6
  Demux1/2 -> Bus Assignment/5
  Demux1/1 -> Bus Assignment/4
  Bus Selector2/1 -> Data Type Conversion5/1
  Bus Selector3/1 -> Subsystem Reference/1
  Bus Selector4/1 -> m/s to cm/s/1

== system Quad_UAV_Dynamics/Plant/Non-Linear Airframe/AC model/Aerodynamic/Drag Calc ==
  Density : Inport  Unit=kg/m^3
  vel : Inport  Port=2  Unit=m/s
  Dynamic Pressure : aerolibasang/Dynamic Pressure
  Heigth : Gain  Gain=0.1
  Mux1 : Mux  Inputs=3
  Product : Product  Inputs=3  RndMeth=Zero
  Square : Math  Operator=square
  diameter : Constant  Value=Vehicle.Airframe.armLength*sqrt(2)  SampleTime=0
  dragCoeff : Constant  Value=Vehicle.Airframe.Cdx  SampleTime=0
  drag : Outport  Unit=N  VectorParamsAs1DForOutWhenUnconnected=off
  wires:
  Product/1 -> drag/1
  dragCoeff/1 -> Product/3  "Cd"
  Dynamic Pressure/1 -> Product/1  "q"
  diameter/1 -> Heigth/1, Square/1
  Mux1/1 -> Product/2  "S"
  Heigth/1 -> Mux1/2, Mux1/1
  vel/1 -> Dynamic Pressure/1
  Density/1 -> Dynamic Pressure/2
  Square/1 -> Mux1/3

== system Quad_UAV_Dynamics/Plant/Non-Linear Airframe/AC model/Ground Model/Friction Force ==
  V : Inport
  Fn : Inport  Port=2
  Product : Product
  Saturation : Saturate  UpperLimit=contact.translation.maxFriction  LowerLimit=-contact.translation.maxFriction
  Soft Coulomb Friction : Subsystem
  Unary Minus : UnaryMinus
  Friction : Outport
  wires:
  Fn/1 -> Product/2
  Soft Coulomb Friction/1(Out1) -> Product/1
  Product/1 -> Unary Minus/1
  V/1 -> Soft Coulomb Friction/1(In1)
  Unary Minus/1 -> Saturation/1
  Saturation/1 -> Friction/1

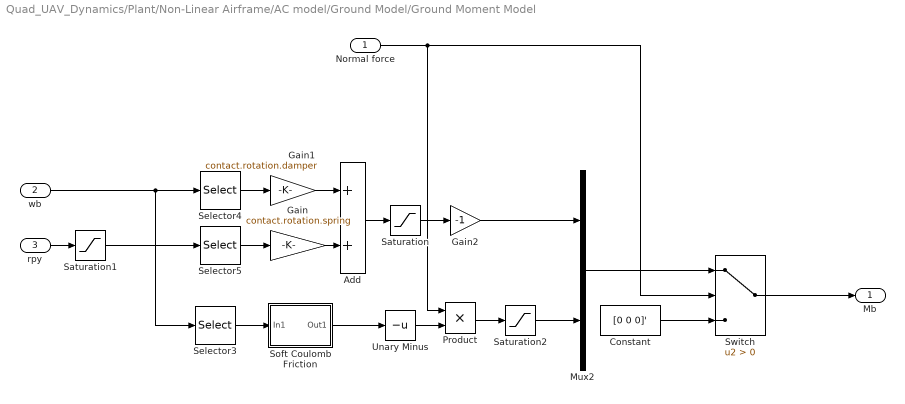
== system Quad_UAV_Dynamics/Plant/Non-Linear Airframe/AC model/Ground Model/Ground Moment Model ==
  Normal force : Inport
  wb : Inport  Port=2
  rpy : Inport  Port=3
  Add : Sum
  Constant : Constant  Value=[0 0 0]'
  Gain : Gain  Gain=contact.rotation.spring
  Gain1 : Gain  Gain=contact.rotation.damper
  Gain2 : Gain  Gain=-1
  Mux2 : Mux  Inputs=2
  Product : Product
  Saturation : Saturate  UpperLimit=control.rotation.maxMoment  LowerLimit=-control.rotation.maxMoment
  Saturation1 : Saturate  UpperLimit=20*pi/180  LowerLimit=-20*pi/180
  Saturation2 : Saturate  UpperLimit=control.rotation.maxMoment  LowerLimit=-control.rotation.maxMoment
  Selector3 : Selector  InputPortWidth=3  IndexOptions=Index vector (dialog)  Indices=[3]  OutputSizes=1
  Selector4 : Selector  InputPortWidth=3  IndexOptions=Index vector (dialog)  Indices=[1, 2]  OutputSizes=1
  Selector5 : Selector  InputPortWidth=3  IndexOptions=Index vector (dialog)  Indices=[1, 2]  OutputSizes=1
  Soft Coulomb Friction : Subsystem
  Switch : Switch  Criteria=u2 > Threshold  SaturateOnIntegerOverflow=off  InputSameDT=off
  Unary Minus : UnaryMinus
  Mb : Outport
  wires:
  Gain2/1 -> Mux2/1
  Add/1 -> Saturation/1
  Gain/1 -> Add/2
  Saturation/1 -> Gain2/1
  Selector4/1 -> Gain1/1
  Gain1/1 -> Add/1
  Constant/1 -> Switch/3
  Selector5/1 -> Gain/1
  Switch/1 -> Mb/1
  Mux2/1 -> Switch/1
  Normal force/1 -> Product/1, Switch/2
  rpy/1 -> Saturation1/1
  Saturation1/1 -> Selector5/1
  wb/1 -> Selector4/1, Selector3/1
  Selector3/1 -> Soft Coulomb Friction/1(In1)
  Soft Coulomb Friction/1(Out1) -> Unary Minus/1
  Unary Minus/1 -> Product/2
  Product/1 -> Saturation2/1
  Saturation2/1 -> Mux2/2

== system Quad_UAV_Dynamics/Plant/Non-Linear Airframe/AC model/Ground Model/Normal Force ==
  Vz : Inport
  Z : Inport  Port=2
  Add : Sum
  Constant : Constant  Value=0
  Damper Kp : Gain  Gain=-contact.translation.damper
  Saturation : Saturate  UpperLimit=contact.translation.maxNormal  LowerLimit=0
  Spring Kp : Gain  Gain=-contact.translation.spring
  Switch : Switch  Criteria=u2 > Threshold  SaturateOnIntegerOverflow=off  InputSameDT=off
  Unary Minus : UnaryMinus
  Unary Minus1 : UnaryMinus
  Normal : Outport
  wires:
  Constant/1 -> Switch/1
  Z/1 -> Unary Minus/1
  Switch/1 -> Saturation/1
  Damper Kp/1 -> Add/2
  Add/1 -> Switch/3
  Spring Kp/1 -> Add/1
  Vz/1 -> Unary Minus1/1
  Saturation/1 -> Normal/1
  Unary Minus/1 -> Spring Kp/1, Switch/2
  Unary Minus1/1 -> Damper Kp/1

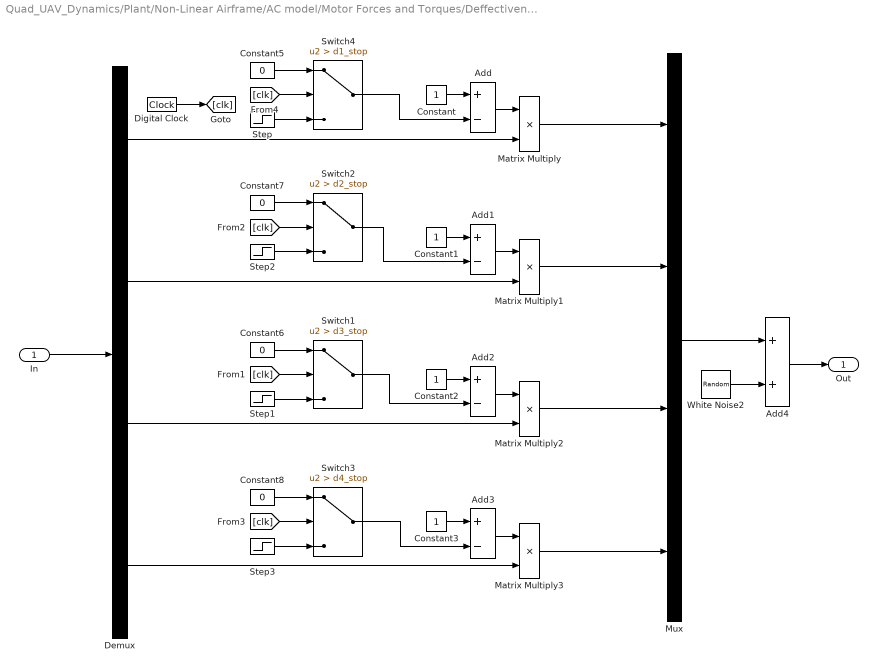
== system Quad_UAV_Dynamics/Plant/Non-Linear Airframe/AC model/Motor Forces and Torques/Deffectiveness ==
  In : Inport
  Add{,1..3} (4 alike) : Sum  Inputs=+-
  Add4 : Sum
  Constant{,1..3} (4 alike) : Constant
  Constant{5..8} (4 alike) : Constant  Value=0
  Demux : Demux
  Digital Clock : DigitalClock  SampleTime=SamplingTime.Ts
  Matrix Multiply{,1..3} (4 alike) : Product
  Mux : Mux
  Step : Step  Time=d1_start  After=d1  SampleTime=0
  Step1 : Step  Time=d3_start  After=d3  SampleTime=0
  Step2 : Step  Time=d2_start  After=d2  SampleTime=0
  Step3 : Step  Time=d4_start  After=d4  SampleTime=0
  Switch1 : Switch  Criteria=u2 > Threshold  Threshold=d3_stop  SaturateOnIntegerOverflow=off  InputSameDT=off
  Switch2 : Switch  Criteria=u2 > Threshold  Threshold=d2_stop  SaturateOnIntegerOverflow=off  InputSameDT=off
  Switch3 : Switch  Criteria=u2 > Threshold  Threshold=d4_stop  SaturateOnIntegerOverflow=off  InputSameDT=off
  Switch4 : Switch  Criteria=u2 > Threshold  Threshold=d1_stop  SaturateOnIntegerOverflow=off  InputSameDT=off
  White Noise2 : RandomNumber  DisableCoverage=on  Variance=diag(Estimator.Q_gamma)  Seed=[23335 23336 23337 23338]
  Out : Outport
  wires:
  Matrix Multiply3/1 -> Mux/4
  Matrix Multiply2/1 -> Mux/3
  Matrix Multiply1/1 -> Mux/2
  Matrix Multiply/1 -> Mux/1
  Constant3/1 -> Add3/1
  Switch3/1 -> Add3/2
  Add3/1 -> Matrix Multiply3/1
  Switch1/1 -> Add2/2
  Constant2/1 -> Add2/1
  Add2/1 -> Matrix Multiply2/1
  Switch2/1 -> Add1/2
  Constant1/1 -> Add1/1
  Add1/1 -> Matrix Multiply1/1
  Constant/1 -> Add/1
  Switch4/1 -> Add/2
  Add/1 -> Matrix Multiply/1
  Demux/4 -> Matrix Multiply3/2
  Demux/3 -> Matrix Multiply2/2
  Demux/2 -> Matrix Multiply1/2
  Demux/1 -> Matrix Multiply/2
  In/1 -> Demux/1
  [clk] -> Switch3/2
  Constant8/1 -> Switch3/1
  Step3/1 -> Switch3/3
  Step2/1 -> Switch2/3
  Constant7/1 -> Switch2/1
  [clk] -> Switch2/2
  [clk] -> Switch1/2
  Constant6/1 -> Switch1/1
  Step1/1 -> Switch1/3
  Step/1 -> Switch4/3
  Constant5/1 -> Switch4/1
  [clk] -> Switch4/2
  Digital Clock/1 -> [clk]
  White Noise2/1 -> Add4/2
  Mux/1 -> Add4/1
  Add4/1 -> Out/1

== system Quad_UAV_Dynamics/Plant/Non-Linear Airframe/AC model/Motor Forces and Torques/Gyroscopic Moments ==
  Omega : Inport
  Gain : Gain  Gain=Vehicle.Motor.hubInertia
  Gain1 : Gain  Gain=-1
  Gyroscopic : Gain  Gain=[1 -1 1 -1]
  Sum of Elements : Sum  Inputs=+
  Vector Concatenate : Concatenate  NumInputs=3
  Zero : Constant  Value=0  OutDataTypeStr=Inherit: Inherit via back propagation
  M : Outport
  wires:
  Vector Concatenate/1 -> M/1
  Zero/1 -> Vector Concatenate/3
  Gain1/1 -> Vector Concatenate/2
  Sum of Elements/1 -> Gain/1
  Gain/1 -> Vector Concatenate/1, Gain1/1
  Omega/1 -> Gyroscopic/1
  Gyroscopic/1 -> Sum of Elements/1

== system Quad_UAV_Dynamics/Plant/Non-Linear Airframe/AC model/Motor Forces and Torques/Motor ==
  PWM : Inport
  Demux : Demux
  Gain1 : Gain  Gain=Vehicle.Motor.maxRPM
  Mux16 : Mux
  Transfer Fcn{1..4} (4 alike) : TransferFcn  Denominator=[1/Vehicle.Motor.Bandwidth 1]
  rpm : Outport
  wires:
  Demux/4 -> Transfer Fcn3/1
  Transfer Fcn1/1 -> Mux16/2
  Transfer Fcn2/1 -> Mux16/3
  Demux/2 -> Transfer Fcn1/1
  Demux/1 -> Transfer Fcn4/1
  Transfer Fcn3/1 -> Mux16/4
  Transfer Fcn4/1 -> Mux16/1
  Demux/3 -> Transfer Fcn2/1
  PWM/1 -> Demux/1
  Mux16/1 -> Gain1/1
  Gain1/1 -> rpm/1

== system Quad_UAV_Dynamics/Plant/Non-Linear Airframe/AC model/Rotor Model/Thrust model ==
  In1 : Inport
  Demux : Demux
  Mux : Mux
  Transfer Fcn{,2..4} (4 alike) : TransferFcn  Numerator=[rotorThrustMax]  Denominator=[rotorTimeConst 1]
  Out1 : Outport
  wires:
  Transfer Fcn3/1 -> Mux/2
  Demux/1 -> Transfer Fcn4/1
  Transfer Fcn2/1 -> Mux/3
  Demux/3 -> Transfer Fcn2/1
  Mux/1 -> Out1/1
  Transfer Fcn4/1 -> Mux/1
  Demux/4 -> Transfer Fcn/1
  Demux/2 -> Transfer Fcn3/1
  Transfer Fcn/1 -> Mux/4
  In1/1 -> Demux/1

== system Quad_UAV_Dynamics/Plant/Non-Linear Airframe/AC model/Rotor Model/Torque model ==
  In1 : Inport
  Demux : Demux
  Mux : Mux
  Transfer Fcn{1..4} (4 alike) : TransferFcn  Numerator=[rotorTorqueMax]  Denominator=[rotorTimeConst 1]
  Out1 : Outport
  wires:
  Transfer Fcn4/1 -> Mux/4
  Demux/1 -> Transfer Fcn1/1
  Transfer Fcn3/1 -> Mux/3
  Transfer Fcn2/1 -> Mux/2
  Demux/2 -> Transfer Fcn2/1
  Demux/4 -> Transfer Fcn4/1
  Demux/3 -> Transfer Fcn3/1
  Mux/1 -> Out1/1
  Transfer Fcn1/1 -> Mux/1
  In1/1 -> Demux/1

== system Quad_UAV_Dynamics/Plant/Non-Linear Airframe/AC model/Ground Model/Friction Force/Soft Coulomb Friction ==
  note: Pennestrì, E., Rossi, V., Salvini, P. et al. Review and comparison of dry friction force models. Nonlinear Dyn 83, 1785–1801 (2016). https://doi.org/10.1007/s11071-015-2485-3
  In1 : Inport
  Tanh : Trigonometry  Operator=tanh
  friction coefficient : Gain  Gain=contact.translation.friction
  vd : Gain  Gain=1/contact.translation.vd
  Out1 : Outport
  wires:
  In1/1 -> vd/1
  vd/1 -> Tanh/1
  Tanh/1 -> friction coefficient/1
  friction coefficient/1 -> Out1/1

== system Quad_UAV_Dynamics/Plant/Non-Linear Airframe/AC model/Ground Model/Ground Moment Model/Soft Coulomb Friction ==
  note: Pennestrì, E., Rossi, V., Salvini, P. et al. Review and comparison of dry friction force models. Nonlinear Dyn 83, 1785–1801 (2016). https://doi.org/10.1007/s11071-015-2485-3
  In1 : Inport
  Tanh : Trigonometry  Operator=tanh
  friction coefficient : Gain  Gain=control.rotation.friction
  vd : Gain  Gain=1/control.rotation.vd
  Out1 : Outport
  wires:
  In1/1 -> vd/1
  vd/1 -> Tanh/1
  Tanh/1 -> friction coefficient/1
  friction coefficient/1 -> Out1/1

== matlab function Quad_UAV_Dynamics/Plant/Non-Linear Airframe/AC model/Rotor Model/MATLAB Function ==
  data: thrustEachRotor input; tauEachRotor input; rotorPositions input; netF output; netM output; rotorDir input
function [netF, netM] = getForceMoment(thrustEachRotor, tauEachRotor, rotorPositions, rotorDir)
%#codegen
Fx = 0;
Fy = 0;
Fz = -sum(thrustEachRotor);

netF = [Fx; Fy; Fz];

netM = [0; 0; 0]; %initialize
    for i = 1:4
        rotPos = rotorPositions(:, i);
        Fi = [0, 0, -thrustEachRotor(i)]';
        netM = netM +  cross(rotPos, Fi);%contribution from thrusts of each propeller
        netM(3) = netM(3) - rotorDir(i)*tauEachRotor(i); %contribution from counter torque acting on propeller
    end

end

== matlab function Quad_UAV_Dynamics/Controller/Position & Altitude controller/Rotation mat  ==
  data: theta input; R output
function R = get_r_mat(theta)
R = [cos(theta) -sin(theta); sin(theta) cos(theta)]';
